simulink model "terrain_test"  (Simulink 7.0)
settings: Solver=ode1  StartTime=0.0  StopTime=inf  FixedStep=0.002  RelTol=1e-3
undefined symbols (not defined in the file or in its folder): Visualization
libraries: quarc_library x3, simulink x1
settings Model: Creator=Derek  LastModifiedBy=Derek  ExtModeTrigDuration=5000
settings SolverCC: PositivePriorityOrder=on
settings RTWCC: SystemTargetFile=quarc_win64.tlc  TemplateMakefile=quarc_default_tmf  Description=QUARC Win64 Target  ProcessScript=quarc_win64_make_rtw_hook
settings STFCustomTargetCC: TargetPreCompLibLocation=C:\PROGRA~3\QUARC\lib\2007b\win64\release  GenFloatMathFcnCalls=ANSI_C  SystemTargetFile=quarc_win64.tlc
settings GRTTargetCC: TargetPreCompLibLocation=C:\PROGRA~3\QUARC\lib\2007b\win64\release  CompOptLevelCompliant=off  MatFileLogging=off  ExtMode=on  ExtModeMexFile=quarc_comm

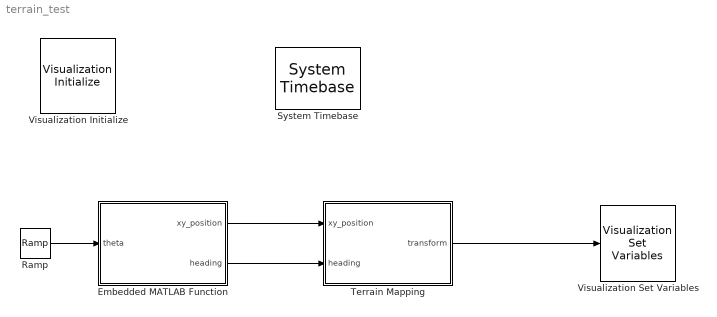
== system terrain_test ==
  Embedded MATLAB Function : Stateflow chart
  Ramp : simulink/Sources/Ramp  SystemSampleTime=-1  slope=0.14  start=0  X0=0
  System Timebase : quarc_library/Advanced/Timing/System Timebase  stop_on_overrun=off
  Terrain Mapping : Stateflow chart
  Visualization Initialize : quarc_library/User Interface/Visualization/Visualization Initialize  object_name=Visualization-1  scene_file=terrain_test.xml  uri={'normal','shmem://%m:2?local=yes';'Configuration','';}  apply_uri_to_all_configs=off  server_send_size=1000000  server_receive_size=1000  derive_from_server=on  client_send_size=1000  client_receive_size=1000000  variables=[ 33 ]  initial_values=single([ 1 0 -0 0 0 1 0 0 0 0 1 0 0 0 0 1 ])  open_on_start=on  close_on_stop=on
      settings: AttributesFormatString=%<object_name>
  Visualization Set Variables : quarc_library/User Interface/Visualization/Visualization Set Variables  object_name=Visualization-1  offset=[ 0 ]  data_type=[ 2 ]  length=[ 16 ]  sample_time=visualization_get_frame_period  actor_name={'actor.box/Transform'}
      settings: AttributesFormatString=(%<object_name>)
  wires:
  Ramp/1 -> Embedded MATLAB Function/1(theta)
  Embedded MATLAB Function/1(xy_position) -> Terrain Mapping/1(xy_position)
  Terrain Mapping/1(transform) -> Visualization Set Variables/1
  Embedded MATLAB Function/2(heading) -> Terrain Mapping/2(heading)

== matlab function Terrain Mapping ==
  data: xy_position input inherited; transform output inherited; heading input inherited
function transform  = fcn(xy_position, heading)
% This block supports the Embedded MATLAB subset.
% See the help menu for details. 


gridx = 200;
gridy = 200;
sizex = 2000;
sizey = 2000;
sizez = 100;

delta = 1;

[rx, ry, z] = calc_surface_angles_pos(xy_position(1), xy_position(2), gridx, gridy, delta, sizex, sizey, sizez);  


rot_x = [1 0 0 0; 0 cos(rx) -sin(rx) 0; 0 sin(rx) cos(rx) 0; 0 0 0 1];
rot_y = [cos(ry) 0 sin(ry) 0; 0 1 0 0; -sin(ry) 0 cos(ry) 0; 0 0 0 1];
rot_z = [cos(heading) -sin(heading) 0 0; sin(heading) cos(heading) 0 0; 0 0 1 0; 0 0 0 1];


position = [1 0 0 xy_position(1); 0 1 0 xy_position(2); 0 0 1 z+2; 0 0 0 1]*rot_x*rot_y*rot_z;

transform = position;
    


function [rx, ry, z] = calc_surface_angles_pos(x, y, gridx, gridy, delta, sizex, sizey, sizez)

z = calc_surface_z(x*gridx/sizex, y*gridy/sizey, gridx, gridy)*sizez; 

zN = calc_surface_z(x*gridx/sizex, (y+delta)*gridy/sizey, gridx, gridy)*sizez; 
zE = calc_surface_z((x+delta)*gridx/sizex, y*gridy/sizey, gridx, gridy)*sizez; 

rx = atan2(zE-z, delta);
ry = atan2(zN-z, delta);

    
    
function z = calc_surface_z(x, y, max_x, max_y)

z = (sin(y*0.1)*sin(x*0.1)*cos(y*0.03) + cos(x*0.3)*sin(y*0.4)*0.1) + 1;
z = z*sigmoid(x, y, max_x, max_y); 
z = z*0.5;

%%
function scale = sigmoid(x,y,max_x,max_y)

%sigmoid parameters

b1x = max_x*0.1;
b2x = max_x - max_x*0.1;

b1y = max_y*0.1;
b2y = max_y - max_y*0.1;


c = 0.1;

scalex = 1./(1+exp(-c.*(x-b1x))) - 1./(1+exp(-c.*(x-b2x)));
scaley = 1./(1+exp(-c.*(y-b1y))) - 1./(1+exp(-c.*(y-b2y)));

scale = scalex*scaley;

== matlab function Embedded MATLAB Function ==
  data: theta input inherited; xy_position output inherited; heading output inherited
function [xy_position, heading] = fcn(theta)
% This block supports the Embedded MATLAB subset.
% See the help menu for details. 


gridx = 200;
gridy = 200;
sizex = 2000;
sizey = 2000;

r = 51;
cx = 100;
cy = 100;

x = cx + (r + 5*sin(2*theta))*cos(theta);
y = cy + (r + 5*sin(4*theta)*sin(theta))*sin(theta);

xy_position = [x/gridx*sizex y/gridy*sizey];


angle = atan2( ...
    (10*cos(2*theta)*cos(theta)-(51+5*sin(2*theta))*sin(theta))*sizex/gridx, ...
    ((20*cos(4*theta)*sin(theta)+5*sin(4*theta)*cos(theta))*sin(theta)+(51+5*sin(4*theta)*sin(theta))*cos(theta))*sizey/gridy ...
    );

heading = -angle+pi/2;
